simulink model "Quiz7Sim2016a"  (R2016a)
settings: Solver=FixedStepAuto  SolverMode=SingleTasking  StartTime=0.0  StopTime=2  FixedStep=1e-4  MaxStep=1e-4  MinStep=1e-4  RelTol=1e-3
libraries: simulink x1
settings Model: Creator=Casper Versteeg  LastModifiedBy=Casper Versteeg
settings DebuggingCC: SFUnexpectedBacktrackingDiag=error  SFNoUnconditionalDefaultTransitionDiag=error
settings GRTTargetCC: TargetLangStandard=C99 (ISO)  GeneratePreprocessorConditionals=Use local settings
settings ConfigComp: CovMetricSettings=dwe  CovHtmlReporting=off  CovSaveCumulativeToWorkspaceVar=off  CovSaveSingleToWorkspaceVar=off  CovExternalEMLEnable=on

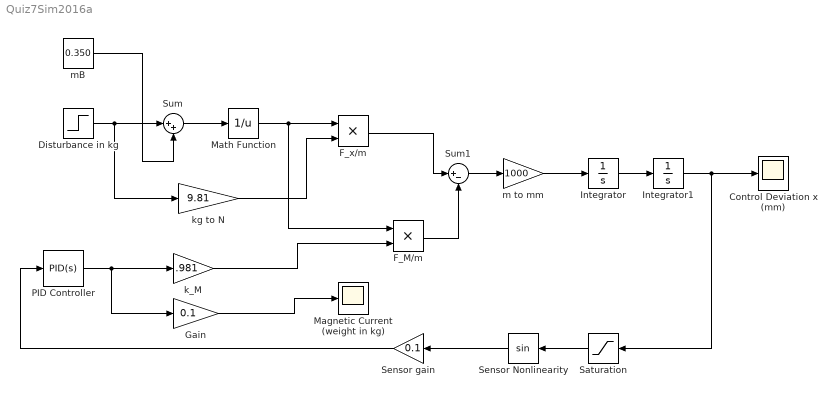
== system Quiz7Sim2016a ==
  Control Deviation x (mm) : Scope
  Disturbance in kg : Step  Time=0  After=0.2  SampleTime=0
  F_M/m : Product
  F_x/m : Product
  Gain : Gain  Gain=0.1
  Integrator : Integrator
  Integrator1 : Integrator
  Magnetic Current (weight in kg) : Scope
  Math Function : Math  Operator=reciprocal  SaturateOnIntegerOverflow=on
  PID Controller : simulink/Continuous/PID Controller  Controller=PID  TimeDomain=Continuous-time  SampleTime=-1  IntegratorMethod=Forward Euler  FilterMethod=Forward Euler  Form=Parallel  UseFilter=on  ControllerParametersSource=internal  P=90  I=0  D=10  N=25000  InitialConditionSource=internal  InitialConditionForIntegrator=0  InitialConditionForFilter=0  ExternalReset=none  LimitOutput=off  UpperSaturationLimit=inf  LowerSaturationLimit=-inf  LinearizeAsGain=on  AntiWindupMode=none  Kb=1  TrackingMode=off  Kt=1  PParamMin=[]  PParamMax=[]  IParamMin=[]  IParamMax=[]  DParamMin=[]  DParamMax=[]  NParamMin=[]  NParamMax=[]  KbParamMin=[]  KbParamMax=[]  KtParamMin=[]  KtParamMax=[]  POutMin=[]  POutMax=[]  IOutMin=[]  IOutMax=[]  DOutMin=[]  DOutMax=[]  NOutMin=[]  NOutMax=[]  KbOutMin=[]  KbOutMax=[]  KtOutMin=[]  KtOutMax=[]  IntegratorOutMin=[]  IntegratorOutMax=[]  FilterOutMin=[]  FilterOutMax=[]  SumOutMin=[]  SumOutMax=[]  SumI1OutMin=[]  SumI1OutMax=[]  SumI2OutMin=[]  SumI2OutMax=[]  SumI3OutMin=[]  SumI3OutMax=[]  SumDOutMin=[]  SumDOutMax=[]  SaturationOutMin=[]  SaturationOutMax=[]  IntegratorContinuousStateAttributes=''  IntegratorStateMustResolveToSignalObject=off  IntegratorRTWStateStorageClass=Auto  FilterContinuousStateAttributes=''  FilterStateMustResolveToSignalObject=off  FilterRTWStateStorageClass=Auto  DifferentiatorICPrevScaledInput=0  DifferentiatorOutMin=[]  DifferentiatorOutMax=[]
  Saturation : Saturate  UpperLimit=0.785  LowerLimit=-0.785
  Sensor Nonlinearity : Trigonometry
  Sensor gain : Gain  Gain=0.1
  Sum : Sum  Inputs=|++
  Sum1 : Sum  Inputs=|+-
  k_M : Gain  Gain=.981
  kg to N : Gain  Gain=9.81
  m to mm : Gain  Gain=1000
  mB : Constant  Value=0.350
  wires:
  mB/1 -> Sum/2
  Disturbance in kg/1 -> kg to N/1, Sum/1
  Sum/1 -> Math Function/1
  kg to N/1 -> F_x/m/2
  Sum1/1 -> m to mm/1
  F_x/m/1 -> Sum1/1
  F_M/m/1 -> Sum1/2
  k_M/1 -> F_M/m/2
  Math Function/1 -> F_x/m/1, F_M/m/1
  m to mm/1 -> Integrator/1
  Integrator/1 -> Integrator1/1
  Integrator1/1 -> Saturation/1, Control Deviation x (mm)/1
  Saturation/1 -> Sensor Nonlinearity/1
  Sensor Nonlinearity/1 -> Sensor gain/1
  Sensor gain/1 -> PID Controller/1
  PID Controller/1 -> Gain/1, k_M/1
  Gain/1 -> Magnetic Current (weight in kg)/1
